simulink model "Amortiguador_simulink"  (R2025b)
settings: Solver=VariableStepAuto  StartTime=0.0  StopTime=20  RelTol=1e-3
settings Model: Creator=leona  LastModifiedBy=leona

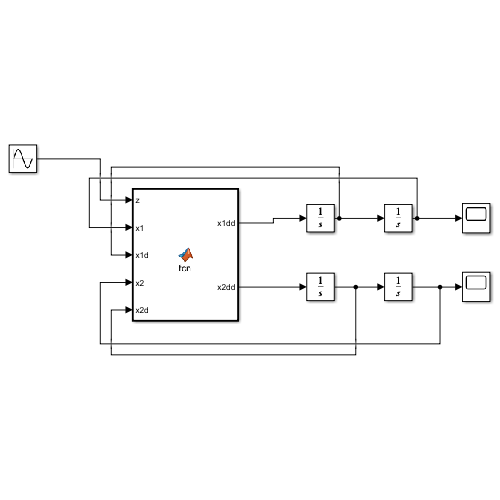
[thumbnail: Simulink's stored preview of the top-level diagram]
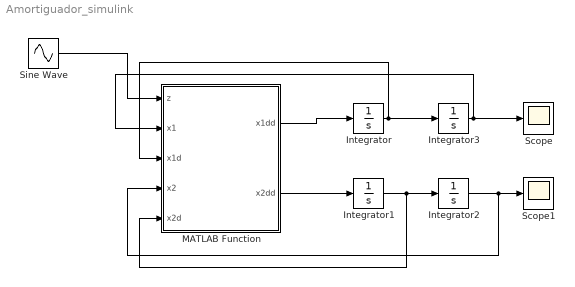
== system Amortiguador_simulink ==
  Integrator{,1..3} (4 alike) : Integrator
  MATLAB Function : MATLAB Function  TreatAsAtomicUnit=on
  Scope : Scope
      settings: ActiveDisplayYMinimum=-0.294332623272251  ActiveDisplayYMaximum=0.21611601712033474
  Scope1 : Scope
      settings: ActiveDisplayYMinimum=-0.29072238808889805  ActiveDisplayYMaximum=0.1765636534368108
  Sine Wave : Sin  Amplitude=0.05  Frequency=0.5*pi  SampleTime=0
  wires:
  MATLAB Function/1(x1dd) -> Integrator/1
  MATLAB Function/2(x2dd) -> Integrator1/1
  Integrator1/1 -> MATLAB Function/5(x2d), Integrator2/1
  Integrator/1 -> MATLAB Function/3(x1d), Integrator3/1
  Integrator3/1 -> MATLAB Function/2(x1), Scope/1
  Integrator2/1 -> MATLAB Function/4(x2), Scope1/1
  Sine Wave/1 -> MATLAB Function/1(z)

== matlab function Amortiguador_simulink/MATLAB Function ==
  data: z input; x1 input; x1d input; x1dd output; x2 input; x2d input; x2dd output
function [x1dd,x2dd] = fcn(z, x1,x1d,x2,x2d)

m1=290;
b1=1000;
m2=59;
k1=16182;
k2=19000;
f=0;

x1dd=(-b1*x1d+b1*x2d-k1*x1+k1*x2+f)/m1;

x2dd=(b1*x1d-b1*x2d+k1*x1-(k1+k2)*x2-f+k2*z)/m2;

end
